simulink subsystem "LMS_adaptiveAlgorithm"  (R2022a)
settings: Solver=VariableStepAuto  StartTime=0.0  StopTime=10.0  RelTol=1e-3
settings Model: Creator=targi  LastModifiedBy=targi

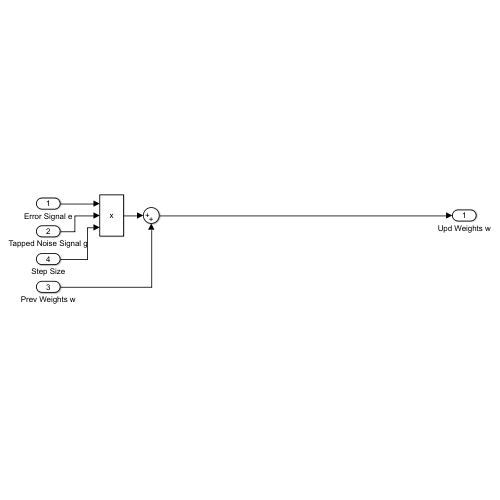
[thumbnail: Simulink's stored preview of the top-level diagram]
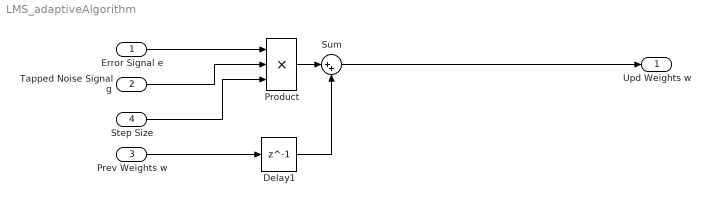
== system LMS_adaptiveAlgorithm ==
  Error Signal e : Inport
  Tapped Noise Signal g : Inport  Port=2
  Prev Weights w : Inport  Port=3
  Step Size : Inport  Port=4
  Delay1 : Delay  DelayLength=1  InitialCondition=0
  Product : Product  Inputs=3
  Sum : Sum  Inputs=|++
  Upd Weights w : Outport
  wires:
  Tapped Noise Signal g/1 -> Product/2
  Step Size/1 -> Product/3
  Product/1 -> Sum/1
  Sum/1 -> Upd Weights w/1
  Prev Weights w/1 -> Delay1/1
  Delay1/1 -> Sum/2
  Error Signal e/1 -> Product/1
